simulink model "inv_pend_losses"  (Simulink 8.2)
settings: Solver=ode45  StartTime=0.0  StopTime=40  RelTol=1e-3
values from neighbouring files (symbols this model uses):
  A = [1 1 ... (first row only)    [execution.m]    (also in lqgcalculation.m = sys.a)
  B = [0 ... (first row only)    [execution.m]    (also in lqgcalculation.m = sys.b)
  h = 0.3    [execution.m]
  K = [20 9]    [execution.m]
settings Model: Creator=mengg_000  LastModifiedBy=Daniel
settings DebuggingCC: InheritedTsInSrcMsg=none

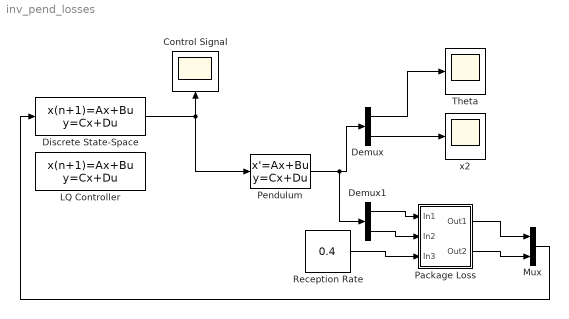
== system inv_pend_losses ==
  Control Signal : Scope
      settings: TimeRange=1  YMin=1  YMax=3.5  SaveName=ry
  Demux : Demux  Outputs=2
  Demux1 : Demux  Outputs=2
  Discrete State-Space : DiscreteStateSpace  A=0  B=[0 0]  C=0  D=-K  SampleTime=h
  LQ Controller : DiscreteStateSpace  A=|  B=|  C="[-12.1798  -13.3262         0]"  D=-8.1263  X0="[0;    0;   0]"  SampleTime=0.02
      A=|
      | [0.0389   -1.5001         0;
      |     0.0828    0.3594         0;
      |   -12.1798  -13.3262         0]
      B=|
      | [ -0.4344;
      |     0.1355;
      |    -8.1263]
  Mux : Mux  Inputs=2
  Package Loss : Subsystem
  "Pendulum " : StateSpace  A=A  B=B  C=eye(2)  D=[0;0]  X0=[0; 0.1]
  Reception Rate : Constant  Value=0.4
  Theta : Scope
      settings: TimeRange=1  YMin=1  YMax=3.5  SaveName=ry1
  x2 : Scope
      settings: TimeRange=1  YMin=1  YMax=3.5  SaveName=ry2
  wires:
  Demux/1 -> Theta/1
  Reception Rate/1 -> Package Loss/3(In3)
  Discrete State-Space/1 -> "Pendulum "/1, Control Signal/1
  "Pendulum "/1 -> Demux1/1, Demux/1
  Demux/2 -> x2/1
  Demux1/2 -> Package Loss/2(In2)
  Demux1/1 -> Package Loss/1(In1)
  Package Loss/2(Out2) -> Mux/2
  Package Loss/1(Out1) -> Mux/1
  Mux/1 -> Discrete State-Space/1

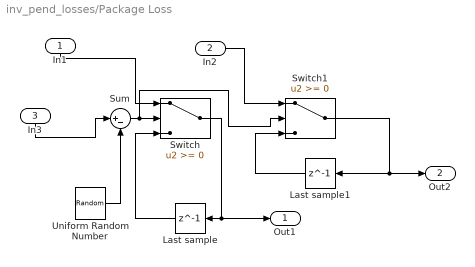
== system inv_pend_losses/Package Loss ==
  In1 : Inport
  In2 : Inport  Port=2
  In3 : Inport  Port=3
  Last sample : Delay  DelayLength=1  SampleTime=h
  Last sample1 : Delay  DelayLength=1  SampleTime=h
  Sum : Sum  Inputs=|+-
  Switch : Switch
  Switch1 : Switch
  Uniform Random Number : UniformRandomNumber  Minimum=0
  Out1 : Outport
  Out2 : Outport  Port=2
  wires:
  Uniform Random Number/1 -> Sum/2
  Sum/1 -> Switch1/2, Switch/2
  In1/1 -> Switch/1
  Switch/1 -> Out1/1, Last sample/1
  Last sample/1 -> Switch/3
  Last sample1/1 -> Switch1/3
  Switch1/1 -> Out2/1, Last sample1/1
  In3/1 -> Sum/1
  In2/1 -> Switch1/1
